simulink model "ordre2ana2 (1)"  (R2014a)
settings: Solver=ode45  StartTime=0.0  StopTime=0.004  FixedStep=Delta  MaxStep=1e-6  RelTol=1e-3
undefined symbols (not defined in the file): Dt, K, tau, Te
settings Model: Creator=aymeric  LastModifiedBy=aymeric

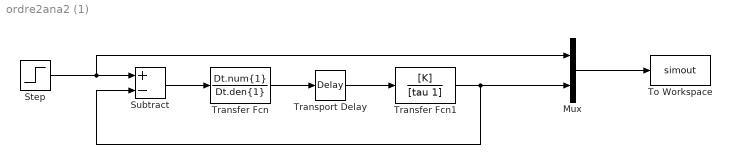
== system ordre2ana2 (1) ==
  Mux : Mux  Inputs=2
  Step : Step  Time=0  SampleTime=0
  Subtract : Sum  Inputs=+-
  To Workspace : ToWorkspace  VariableName=simout  SaveFormat=Timeseries  SampleTime=-1
  Transfer Fcn : TransferFcn  Numerator=Dt.num{1}  Denominator=Dt.den{1}
  Transfer Fcn1 : TransferFcn  Numerator=[K]  Denominator=[tau 1]
  Transport Delay : TransportDelay  DelayTime=Te/2
  wires:
  Step/1 -> Mux/1, Subtract/1
  Mux/1 -> To Workspace/1
  Transport Delay/1 -> Transfer Fcn1/1
  Transfer Fcn1/1 -> Subtract/2, Mux/2
  Subtract/1 -> Transfer Fcn/1
  Transfer Fcn/1 -> Transport Delay/1
